simulink library "sm_motor_grader_lib"  (R2026a)
settings: Solver=VariableStepAuto
undefined symbols (not defined in the file): activeTestCmds, Art, Center, Circle, Driver, HMPST, LiftL, LiftR, LnL, LnR, Loads, Maneuver, motGradParams, Pin, RFL, RFR, RRL, RRR, SceneData, Side, Sphere, StrL, StrR, Tilt, X, Y, Z
libraries: sm_lib x219, nesl_utility x134, fl_lib x53, $bdroot x24, cvt_powertrain_lib x6, simulink_extras x5, grid_element x4, simulink x3, cvt_powertrain_lib_vnts x3, Driver_Long_Lat_Stanley x1, Maneuver_Get_Pose x1, SignalEditorBlockLib x1
(part 2 of 13)

== system sm_motor_grader_lib/Control ==
  m : Inport
  1-D Lookup Table : Lookup_n-D  NumberOfTableDimensions=1  BreakpointsForDimension1=activeTestCmds.get('pArtic').Time  Table=activeTestCmds.get('pArtic').Data  InternalRulePriority=Speed  RndMeth=Simplest
  1-D Lookup Table1 : Lookup_n-D  NumberOfTableDimensions=1  BreakpointsForDimension1=activeTestCmds.get('nHoleLink').Time  Table=activeTestCmds.get('nHoleLink').Data  InternalRulePriority=Speed  RndMeth=Simplest
  1-D Lookup Table10 : Lookup_n-D  NumberOfTableDimensions=1  BreakpointsForDimension1=activeTestCmds.get('qCircle').Time  Table=activeTestCmds.get('qCircle').Data  InternalRulePriority=Speed  RndMeth=Simplest
  1-D Lookup Table11 : Lookup_n-D  NumberOfTableDimensions=1  BreakpointsForDimension1=activeTestCmds.get('mLiftL').Time  Table=activeTestCmds.get('mLiftL').Data  InternalRulePriority=Speed  RndMeth=Simplest
  1-D Lookup Table12 : Lookup_n-D  NumberOfTableDimensions=1  BreakpointsForDimension1=activeTestCmds.get('pPin').Time  Table=activeTestCmds.get('pPin').Data  InternalRulePriority=Speed  RndMeth=Simplest
  1-D Lookup Table13 : Lookup_n-D  NumberOfTableDimensions=1  BreakpointsForDimension1=activeTestCmds.get('mLiftR').Time  Table=activeTestCmds.get('mLiftR').Data  InternalRulePriority=Speed  RndMeth=Simplest
  1-D Lookup Table2 : Lookup_n-D  NumberOfTableDimensions=1  BreakpointsForDimension1=activeTestCmds.get('vVeh').Time  Table=activeTestCmds.get('vVeh').Data  InternalRulePriority=Speed  RndMeth=Simplest
  1-D Lookup Table3 : Lookup_n-D  NumberOfTableDimensions=1  BreakpointsForDimension1=activeTestCmds.get('pSteer').Time  Table=activeTestCmds.get('pSteer').Data  InternalRulePriority=Speed  RndMeth=Simplest
  1-D Lookup Table4 : Lookup_n-D  NumberOfTableDimensions=1  BreakpointsForDimension1=activeTestCmds.get('pLean').Time  Table=activeTestCmds.get('pLean').Data  InternalRulePriority=Speed  RndMeth=Simplest
  1-D Lookup Table5 : Lookup_n-D  NumberOfTableDimensions=1  BreakpointsForDimension1=activeTestCmds.get('pLiftL').Time  Table=activeTestCmds.get('pLiftL').Data  InternalRulePriority=Speed  RndMeth=Simplest
  1-D Lookup Table6 : Lookup_n-D  NumberOfTableDimensions=1  BreakpointsForDimension1=activeTestCmds.get('pLiftR').Time  Table=activeTestCmds.get('pLiftR').Data  InternalRulePriority=Speed  RndMeth=Simplest
  1-D Lookup Table7 : Lookup_n-D  NumberOfTableDimensions=1  BreakpointsForDimension1=activeTestCmds.get('pCircleShift').Time  Table=activeTestCmds.get('pCircleShift').Data  InternalRulePriority=Speed  RndMeth=Simplest
  1-D Lookup Table8 : Lookup_n-D  NumberOfTableDimensions=1  BreakpointsForDimension1=activeTestCmds.get('pTilt').Time  Table=activeTestCmds.get('pTilt').Data  InternalRulePriority=Speed  RndMeth=Simplest
  1-D Lookup Table9 : Lookup_n-D  NumberOfTableDimensions=1  BreakpointsForDimension1=activeTestCmds.get('pShift').Time  Table=activeTestCmds.get('pShift').Data  InternalRulePriority=Speed  RndMeth=Simplest
  Bus Creator : BusCreator  Inputs=14
  Bus Selector : BusSelector  OutputSignals=aSteerWheel
  Clock : Clock
  Closed Loop : Subsystem  VariantControl=Closed_Loop
  Steer Wheel to Cyl Ext : Subsystem
  Terminator2 : Terminator
  Test : Outport
  wires:
  m/1 -> Closed Loop/1(VehBus)
  Closed Loop/1(DrvBus) -> Bus Selector/1
  1-D Lookup Table7/1 -> Bus Creator/7  "pCircleShift"
  1-D Lookup Table/1 -> Bus Creator/2, Steer Wheel to Cyl Ext/2(pArtic)  "pArtic"
  1-D Lookup Table1/1 -> Bus Creator/12  "nHoleLink"
  1-D Lookup Table9/1 -> Bus Creator/10  "pShift"
  1-D Lookup Table2/1 -> Bus Creator/1  "vVeh"
  1-D Lookup Table8/1 -> Bus Creator/9  "pTilt"
  1-D Lookup Table12/1 -> Bus Creator/11  "pPin"
  1-D Lookup Table4/1 -> Bus Creator/4  "pLean"
  1-D Lookup Table6/1 -> Bus Creator/6  "pLiftR"
  Clock/1 -> 1-D Lookup Table/1, 1-D Lookup Table3/1, 1-D Lookup Table6/1, 1-D Lookup Table7/1, 1-D Lookup Table10/1, 1-D Lookup Table8/1, 1-D Lookup Table12/1, 1-D Lookup Table13/1, 1-D Lookup Table11/1, 1-D Lookup Table1/1, 1-D Lookup Table9/1, 1-D Lookup Table5/1, 1-D Lookup Table4/1, 1-D Lookup Table2/1
  Bus Creator/1 -> Test/1
  1-D Lookup Table10/1 -> Bus Creator/8  "qCircle"
  1-D Lookup Table5/1 -> Bus Creator/5  "pLiftL"
  Bus Selector/1 -> Steer Wheel to Cyl Ext/1(qSteer)  "<aSteerWheel>"
  Steer Wheel to Cyl Ext/1(pSteer) -> Bus Creator/3  "pSteer"
  1-D Lookup Table3/1 -> Terminator2/1  "pSteer"
  1-D Lookup Table11/1 -> Bus Creator/13  "mLiftL"
  1-D Lookup Table13/1 -> Bus Creator/14  "mLiftR"

== system sm_motor_grader_lib/Dashboard Input ==
  In : Inport
  Rate Limiter : RateLimiter  RisingSlewLimit=abs((upper_bound-lower_bound)/5)  FallingSlewLimit=-abs((upper_bound-lower_bound)/5)  SampleTimeMode=inherited  InitialCondition=U0
  Saturation : Saturate  UpperLimit=upper_bound  LowerLimit=lower_bound  ZeroCross=off
  Transfer Fcn (with initial outputs) : simulink_extras/Additional Linear/Transfer Fcn (with initial outputs)  N=[1]  D="[tfilt  1]"  Y0=U0  U0=U0
  out : Outport
  wires:
  In/1 -> Saturation/1
  Transfer Fcn (with initial outputs)/1 -> Rate Limiter/1
  Saturation/1 -> Transfer Fcn (with initial outputs)/1
  Rate Limiter/1 -> out/1

== system sm_motor_grader_lib/Data ==
  note: Easy way to create structure for simulation data.
  m : Inport
  1-D Lookup Table : Lookup_n-D  NumberOfTableDimensions=1  BreakpointsForDimension1=activeTestCmds.get('pArtic').Time  Table=activeTestCmds.get('pArtic').Data  InternalRulePriority=Speed  RndMeth=Simplest
  1-D Lookup Table1 : Lookup_n-D  NumberOfTableDimensions=1  BreakpointsForDimension1=activeTestCmds.get('nHoleLink').Time  Table=activeTestCmds.get('nHoleLink').Data  InternalRulePriority=Speed  RndMeth=Simplest
  1-D Lookup Table10 : Lookup_n-D  NumberOfTableDimensions=1  BreakpointsForDimension1=activeTestCmds.get('qCircle').Time  Table=activeTestCmds.get('qCircle').Data  InternalRulePriority=Speed  RndMeth=Simplest
  1-D Lookup Table11 : Lookup_n-D  NumberOfTableDimensions=1  BreakpointsForDimension1=activeTestCmds.get('mLiftL').Time  Table=activeTestCmds.get('mLiftL').Data  InternalRulePriority=Speed  RndMeth=Simplest
  1-D Lookup Table12 : Lookup_n-D  NumberOfTableDimensions=1  BreakpointsForDimension1=activeTestCmds.get('pPin').Time  Table=activeTestCmds.get('pPin').Data  InternalRulePriority=Speed  RndMeth=Simplest
  1-D Lookup Table13 : Lookup_n-D  NumberOfTableDimensions=1  BreakpointsForDimension1=activeTestCmds.get('mLiftR').Time  Table=activeTestCmds.get('mLiftR').Data  InternalRulePriority=Speed  RndMeth=Simplest
  1-D Lookup Table2 : Lookup_n-D  NumberOfTableDimensions=1  BreakpointsForDimension1=activeTestCmds.get('vVeh').Time  Table=activeTestCmds.get('vVeh').Data  InternalRulePriority=Speed  RndMeth=Simplest
  1-D Lookup Table3 : Lookup_n-D  NumberOfTableDimensions=1  BreakpointsForDimension1=activeTestCmds.get('pSteer').Time  Table=activeTestCmds.get('pSteer').Data  InternalRulePriority=Speed  RndMeth=Simplest
  1-D Lookup Table4 : Lookup_n-D  NumberOfTableDimensions=1  BreakpointsForDimension1=activeTestCmds.get('pLean').Time  Table=activeTestCmds.get('pLean').Data  InternalRulePriority=Speed  RndMeth=Simplest
  1-D Lookup Table5 : Lookup_n-D  NumberOfTableDimensions=1  BreakpointsForDimension1=activeTestCmds.get('pLiftL').Time  Table=activeTestCmds.get('pLiftL').Data  InternalRulePriority=Speed  RndMeth=Simplest
  1-D Lookup Table6 : Lookup_n-D  NumberOfTableDimensions=1  BreakpointsForDimension1=activeTestCmds.get('pLiftR').Time  Table=activeTestCmds.get('pLiftR').Data  InternalRulePriority=Speed  RndMeth=Simplest
  1-D Lookup Table7 : Lookup_n-D  NumberOfTableDimensions=1  BreakpointsForDimension1=activeTestCmds.get('pCircleShift').Time  Table=activeTestCmds.get('pCircleShift').Data  InternalRulePriority=Speed  RndMeth=Simplest
  1-D Lookup Table8 : Lookup_n-D  NumberOfTableDimensions=1  BreakpointsForDimension1=activeTestCmds.get('pTilt').Time  Table=activeTestCmds.get('pTilt').Data  InternalRulePriority=Speed  RndMeth=Simplest
  1-D Lookup Table9 : Lookup_n-D  NumberOfTableDimensions=1  BreakpointsForDimension1=activeTestCmds.get('pShift').Time  Table=activeTestCmds.get('pShift').Data  InternalRulePriority=Speed  RndMeth=Simplest
  Bus Creator : BusCreator  Inputs=14
  Clock : Clock
  Signal Editor : SignalEditorBlockLib/Signal Editor  Commented=on  FileName=MotGradTestCommands.mat  ActiveScenario=TestCmds  ActiveSignal=nHoleLink  IsBus=off  OutputBusObjectStr=Bus: BusObject  SampleTime=0  Interpolate=off  ZeroCross=off  OutputAfterFinalValue=Setting to zero  Unit=inherit  PreserveSignalName=on  ApplySigPropsToAllScenarios=on  ApplySigPropsToAllSignals=off  SignalPropertySource=Dialog parameters
  Terminator : Terminator
  Transfer Fcn : TransferFcn  Denominator=[0.1 1]
  Test : Outport
  wires:
  Clock/1 -> 1-D Lookup Table9/1, 1-D Lookup Table12/1, 1-D Lookup Table13/1, 1-D Lookup Table11/1, 1-D Lookup Table1/1, 1-D Lookup Table8/1, 1-D Lookup Table10/1, 1-D Lookup Table7/1, 1-D Lookup Table6/1, 1-D Lookup Table5/1, 1-D Lookup Table4/1, 1-D Lookup Table3/1, 1-D Lookup Table/1, 1-D Lookup Table2/1
  1-D Lookup Table7/1 -> Bus Creator/7  "pCircleShift"
  1-D Lookup Table10/1 -> Bus Creator/8  "qCircle"
  1-D Lookup Table12/1 -> Bus Creator/11  "pPin"
  1-D Lookup Table1/1 -> Bus Creator/12  "nHoleLink"
  1-D Lookup Table4/1 -> Bus Creator/4  "pLean"
  1-D Lookup Table/1 -> Bus Creator/2  "pArtic"
  1-D Lookup Table5/1 -> Bus Creator/5  "pLiftL"
  1-D Lookup Table8/1 -> Bus Creator/9  "pTilt"
  1-D Lookup Table9/1 -> Bus Creator/10  "pShift"
  1-D Lookup Table3/1 -> Bus Creator/3  "pSteer"
  1-D Lookup Table6/1 -> Bus Creator/6  "pLiftR"
  Transfer Fcn/1 -> Bus Creator/1  "vVeh"
  Bus Creator/1 -> Test/1
  m/1 -> Terminator/1
  1-D Lookup Table11/1 -> Bus Creator/13  "mLiftL"
  1-D Lookup Table13/1 -> Bus Creator/14  "mLiftR"
  1-D Lookup Table2/1 -> Transfer Fcn/1  "vVeh"

== system sm_motor_grader_lib/Drawbar ==
  Bus Element In : Inport  PortName=cmd  Element=qCircle
  Actuator : Subsystem  Variant=on  VariantControlMode=label  VariantControl=Position  LabelModeActiveChoice=Position
      settings: AttributesFormatString=%<LabelModeActiveChoice>
  Common Gear Constraint : sm_lib/Gears and Couplings/Gears/Common Gear Constraint  GearType=Internal  SpecificationType=CenterDistanceRatio  CenterDistance=0.439843707288225  CenterDistanceUnits=m  GearRatio=25/3  BaseGearRadius=1  BaseGearRadiusUnits=m  FollGearRadius=1  FollGearRadiusUnits=m  SensingForceTorqueDirection=FollowerOnBase  SensingForceTorqueResolutionFrame=BaseFrame  SenseForce=off  SenseTorque=off
  Drawbar : Subsystem
      settings: PortSchema="{\"entries\":[{\"content\":{\"sides\":[{\"content\":{\"connectorIds\":[\"LConn1\",\"LConn2\",\"LConn3\"]},\"type\":\"ConnectorPlacement.EquallySpacedRectSide\",\"uuid\":\"c5f191b1-521e-4128-9ed3-e7d77db4b9ac\"},{\"content\":{\"connectorIds\":[\"RConn1\"],\"side\":\"RIGHT\"},\"type\":\"ConnectorPlacement.EquallySpacedRectSide\",\"uuid\":\"8d32ccf5-09eb-45be-b318-439daa2ebdec\"},{\"content\":{\"connectorIds\":[\"LConn4\",\"LConn5\"],\"side\":\"TOP\"},\"type\":\"ConnectorPlacement.EquallySpacedRectSide\",\"uuid\":\"7fd453ba-2af2-4d29-90fe-6a5fb43a17e4\"}]},\"type\":\"ConnectorPlacement.EquallySpacedConnector\",\"uuid\":\"3987b159-0399-4627-a491-adadc6044e15\"}],\"packageUris\":[\"http://schema.mathworks.com/mf0/Connector/R2020b\"],\"version\":\"1.0\"}"
      mask Display: image('sm_motor_grader_drawbar_IMAGE.png')
  Gain1 : Gain  Gain=motGradParams.circleRot.gearRatio
  Pinion Gear : Subsystem
      settings: PortSchema="{\"entries\":[{\"content\":{\"sides\":[{\"content\":{},\"type\":\"ConnectorPlacement.EquallySpacedRectSide\",\"uuid\":\"c603bcd7-3b50-4fd0-b707-575b3b9ab760\"},{\"content\":{\"connectorIds\":[\"RConn1\"],\"side\":\"RIGHT\"},\"type\":\"ConnectorPlacement.EquallySpacedRectSide\",\"uuid\":\"75766ee4-4855-409c-acb4-47e2457aa3e0\"},{\"content\":{\"connectorIds\":[\"LConn1\"],\"side\":\"TOP\"},\"type\":\"ConnectorPlacement.EquallySpacedRectSide\",\"uuid\":\"8e8e6d6f-405e-48e3-9dc6-817f2641e967\"}]},\"type\":\"ConnectorPlacement.EquallySpacedConnector\",\"uuid\":\"69d12768-35c2-4c56-b984-34512094e0a2\"}],\"packageUris\":[\"http://schema.mathworks.com/mf0/Connector/R2020b\"],\"version\":\"1.0\"}"
      mask Display: image('sm_motor_grader_pinion_IMAGE.png')
  Revolute Circle : Subsystem
  Spherical Frame : sm_lib/Joints/Spherical Joint  JointMode=Normal  CompositeWrenchDir=FollowerOnBase  CompositeWrenchFrame=BaseFrame  SenseConstraintForce=off  SenseConstraintTorque=off  SenseTotalForce=off  SenseTotalTorque=off  PositionTargetSpecify=on  PositionTargetPriority=Low  PositionTargetRotationMethod=AlignedAxes  PositionTargetFollAlignAxisA=+X  PositionTargetBaseAlignAxisA=+X  PositionTargetFollAlignAxisB=+Y  PositionTargetBaseAlignAxisB=+Y  PositionTargetRotationStandardAxis=+Z  PositionTargetRotationAngle=0  PositionTargetRotationAngleUnits=deg  PositionTargetRotationArbitraryAxis=[0 0 1]  PositionTargetRotationSequenceAxes=FollowerAxes  PositionTargetRotationSequence=XYX  PositionTargetRotationSequenceAngles=[0 0 0]  PositionTargetRotationSequenceAnglesUnits=deg  PositionTargetRotationMatrix=[1 0 0;0 1 0;0 0 1]  PositionTargetQuaternion=[1 0 0 0]  VelocityTargetSpecify=off  VelocityTargetPriority=High  VelocityTargetValue=[0 0 0]  VelocityTargetValueUnits=deg/s  VelocityTargetInFollowerFrame=on  EqPosRotationMethod=None  EqPosFollAlignAxisA=+X  EqPosBaseAlignAxisA=+Y  EqPosFollAlignAxisB=+Y  EqPosBaseAlignAxisB=+Z  EqPosRotationStandardAxis=+Z  EqPosRotationAngle=0  EqPosRotationAngleUnits=deg  EqPosRotationArbitraryAxis=[0 0 1]  EqPosRotationSequenceAxes=FollowerAxes  EqPosRotationSequence=XYX  EqPosRotationSequenceAngles=[0 0 0]  EqPosRotationSequenceAnglesUnits=deg  EqPosRotationMatrix=[1 0 0;0 1 0;0 0 1]  EqPosQuaternion=[1 0 0 0]  SpringStiffness=0  SpringStiffnessUnits=N*m/deg  DampingCoefficient=motGradParams.sphDampingCoeff  DampingCoefficientUnits=N*m/(deg/s)  LowerLimitSpecify=off  LowerLimitBound=15  LowerLimitBoundUnits=deg  LowerLimitStiffness=1e4  LowerLimitStiffnessUnits=N*m/deg  LowerLimitDamping=10  LowerLimitDampingUnits=N*m/(deg/s)  LowerLimitTransitionRegionWidth=0.1  LowerLimitTransitionRegionWidthUnits=deg  UpperLimitSpecify=off  UpperLimitBound=45  UpperLimitBoundUnits=deg  UpperLimitStiffness=1e4  UpperLimitStiffnessUnits=N*m/deg  UpperLimitDamping=10  UpperLimitDampingUnits=N*m/(deg/s)  UpperLimitTransitionRegionWidth=0.1  UpperLimitTransitionRegionWidthUnits=deg  TorqueActuationMode=NoTorque  ActuateTorqueX=off  ActuateTorqueY=off  ActuateTorqueZ=off  ActuateTorque=off  ActuationFrame=BaseFrame  SensePosition=off  SenseVelocityX=off  SenseVelocityY=off  SenseVelocityZ=off  SenseVelocity=off  SenseAccelerationX=off  SenseAccelerationY=off  SenseAccelerationZ=off  SenseAcceleration=off  SenseLowerLimitTorqueMag=off  SenseUpperLimitTorqueMag=off  SensingFrame=BaseFrame
  LiftL : PMIOPort  Side=Left
  LiftR : PMIOPort  Port=2  Side=Left
  Shift : PMIOPort  Port=3  Side=Left
  Frame : PMIOPort  Port=4  Side=Right
  Circle : PMIOPort  Port=5  Side=Right
  Pinion : PMIOPort  Port=6  Side=Right
  Out Bus Element : Outport  PortName=m  Element=Circle
  Out Bus Element1 : Outport  PortName=m  Element=Pinion
  wires:
  Bus Element In/1 -> Gain1/1
  Gain1/1 -> Actuator/1(q)
  Revolute Circle/1(m) -> Out Bus Element/1
  Actuator/1(m) -> Out Bus Element1/1
  connections:
  Frame/RConn1 -- Spherical Frame/LConn1
  Circle/RConn1 -- Common Gear Constraint/RConn1 -- Revolute Circle/RConn1
  Drawbar/LConn1 -- LiftL/RConn1
  Drawbar/LConn2 -- LiftR/RConn1
  Common Gear Constraint/LConn1 -- Pinion Gear/LConn1
  Actuator/RConn1 -- Pinion Gear/RConn1
  Pinion/RConn1 -- Actuator/LConn1
  Spherical Frame/RConn1 -- Drawbar/RConn1
  Revolute Circle/LConn1 -- Drawbar/LConn4
  Actuator/LConn2 -- Drawbar/LConn5
  Drawbar/LConn3 -- Shift/RConn1

== system sm_motor_grader_lib/Frame ==
  In Bus Element : Inport  PortName=cmd  Element=pPin
  Cab : Subsystem
      mask Display: image('sm_motor_grader_cab_IMAGE.png');
  Frame : Subsystem
      settings: PortSchema="{\"entries\":[{\"content\":{\"sides\":[{\"content\":{\"connectorIds\":[\"LConn1\",\"LConn2\",\"LConn3\"]},\"type\":\"ConnectorPlacement.EquallySpacedRectSide\",\"uuid\":\"3cc43cc8-f8b0-4e6c-bbf8-06577467423e\"},{\"content\":{\"connectorIds\":[\"RConn1\",\"RConn2\"],\"side\":\"RIGHT\"},\"type\":\"ConnectorPlacement.EquallySpacedRectSide\",\"uuid\":\"5e6794d0-63d3-423d-8b5c-0e3a6a58fbdc\"},{\"content\":{\"side\":\"TOP\"},\"type\":\"ConnectorPlacement.EquallySpacedRectSide\",\"uuid\":\"99c0f23c-f1a6-459b-839b-cf88b9a4fb05\"},{\"content\":{\"connectorIds\":[\"RConn3\",\"RConn4\",\"RConn5\"],\"side\":\"BOTTOM\"},\"type\":\"ConnectorPlacement.EquallySpacedRectSide\",\"uuid\":\"a57f33c3-f8fe-450e-b3de-9550f46fa3b6\"}]},\"type\":\"ConnectorPlacement.EquallySpacedConnector\",\"uuid\":\"81d8b758-f28c-4ca7-b27e-39357bec09b0\"}],\"packageUris\":[\"http://schema.mathworks.com/mf0/Connector/R2020b\"],\"version\":\"1.0\"}"
      mask Display: image('sm_motor_grader_frame_IMAGE.png')
  Prismatic Joint : sm_lib/Joints/Prismatic Joint  JointMode=Normal  CompositeWrenchDir=FollowerOnBase  CompositeWrenchFrame=BaseFrame  SenseConstraintForce=off  SenseConstraintTorque=off  SenseTotalForce=off  SenseTotalTorque=off  PositionTargetSpecify=off  PositionTargetPriority=High  PositionTargetValue=0  PositionTargetValueUnits=m  VelocityTargetSpecify=off  VelocityTargetPriority=High  VelocityTargetValue=0  VelocityTargetValueUnits=m/s  EquilibriumPosition=0  EquilibriumPositionUnits=m  SpringStiffness=0  SpringStiffnessUnits=N/m  DampingCoefficient=0  DampingCoefficientUnits=N/(m/s)  LowerLimitSpecify=off  LowerLimitBound=-0.1  LowerLimitBoundUnits=m  LowerLimitStiffness=1e2  LowerLimitStiffnessUnits=N/m  LowerLimitDamping=1e1  LowerLimitDampingUnits=N/(m/s)  LowerLimitTransitionRegionWidth=1e-2  LowerLimitTransitionRegionWidthUnits=m  UpperLimitSpecify=off  UpperLimitBound=0  UpperLimitBoundUnits=m  UpperLimitStiffness=1e2  UpperLimitStiffnessUnits=N/m  UpperLimitDamping=1e1  UpperLimitDampingUnits=N/(m/s)  UpperLimitTransitionRegionWidth=1e-2  UpperLimitTransitionRegionWidthUnits=m  TorqueActuationMode=ComputedTorque  MotionActuationMode=InputMotion  SensePosition=off  SenseVelocity=off  SenseAcceleration=off  SenseTorqueForce=off  SenseLowerLimitTorqueForce=off  SenseUpperLimitTorqueForce=off
  SaddlePinSolid : sm_lib/Body Elements/File Solid  ExtGeomFileName=SaddlePin.step  UnitType=FromFile  ExtGeomFileUnits=m  StepReaderType=HEX  ExportConvexHullGeometry=off  InertiaType=CalculateFromGeometry  BasedOnType=Mass  Density=1000  DensityUnits=kg/m^3  Mass=motGradParams.saddlePin.mass  MassUnits=kg  CenterOfMass=[0 0 0]  CenterOfMassUnits=m  MomentsOfInertia=[1 1 1]  MomentsOfInertiaUnits=kg*m^2  ProductsOfInertia=[0 0 0]  ProductsOfInertiaUnits=kg*m^2  GraphicType=FromGeometry  MarkerShape=Sphere  MarkerSize=10  GraphicVisPropType=SimpleVisualProperties  GraphicDiffuseColor=mtrgrd.clr.saddle_pin  GraphicOpacity=1  GraphicSpecularColor=[0.5 0.5 0.5 1.0]  GraphicAmbientColor=[0.15 0.15 0.15 1.0]  GraphicEmissiveColor=[0.0 0.0 0.0 1.0]  GraphicShininess=75  DoExposeReferenceFrame=off  SerializedFrames=<Frames><Frame><Id>Frame1</Id><Value><Name>MainFrame</Name><Origin><Source>GeometricFeature</Source><FeatureName>circular curve 2</FeatureName></Origin><PrimaryAxis><DefinedDirection>+Z</DefinedDirection><Source>GeometricFeature</Source><SourceDirection>+Z</SourceDirection><FeatureName>segment 1</FeatureName></PrimaryAxis><SecondaryAxis><DefinedDirection>+X</DefinedDirection><Source>ReferenceFrame</Source><SourceDirection>+X</SourceDirection><FeatureName></FeatureName></SecondaryAxis></Value></Frame><Frame><Id>Frame2</Id><Value><Name>LinkBar</Name><Origin><Source>GeometricFeature</Source><FeatureName>circular curve 4</FeatureName></Origin><PrimaryAxis><DefinedDirection>+Z</DefinedDirection><Source>GeometricFeature</Source><SourceDirection>+Z</SourceDirection><FeatureName>segment 1</FeatureName></PrimaryAxis><SecondaryAxis><DefinedDirection>+X</DefinedDirection><Source>ReferenceFrame</Source><SourceDirection>+X</SourceDirection><FeatureName></FeatureName></SecondaryAxis></Value></Frame></Frames>
  Simulink-PS Converter : nesl_utility/Simulink-PS Converter  PhysicalDomain=network_engine_domain  SubClassName=ps_input  LeftPortType=input  RightPortType=output  PseudoPeriodic=off  Frequencies=[]  NoiseDistribution=none  NoiseParameters=[]  Unit=m  AffineConversion=off  FilteringAndDerivatives=filter  SimscapeFilterOrder=2  InputFilterTimeConstant=0.001  UdotUserProvided=0
  Cyl : PMIOPort  Side=Left
  R : PMIOPort  Port=2  Side=Left
  F : PMIOPort  Port=3  Side=Right
  Drawbar : PMIOPort  Port=4  Side=Right
  SaddleL : PMIOPort  Port=5  Side=Right
  LinkBar : PMIOPort  Port=6  Side=Right
  SaddleR : PMIOPort  Port=7  Side=Right
  LinkBar1 : PMIOPort  Port=8  Side=Right
  LinkBar2 : PMIOPort  Port=9  Side=Right
  LinkBar3 : PMIOPort  Port=10  Side=Right
  wires:
  In Bus Element/1 -> Simulink-PS Converter/1
  connections:
  LinkBar/RConn1 -- LinkBar1/RConn1 -- LinkBar2/RConn1 -- LinkBar3/RConn1 -- SaddlePinSolid/RConn1
  SaddlePinSolid/LConn1 -- Prismatic Joint/RConn1
  Simulink-PS Converter/RConn1 -- Prismatic Joint/LConn2
  Drawbar/RConn1 -- Frame/RConn1
  Frame/RConn2 -- F/RConn1
  Frame/LConn2 -- Cyl/RConn1
  R/RConn1 -- Frame/LConn3
  Cab/RConn1 -- Frame/LConn1
  Frame/RConn3 -- SaddleL/RConn1
  SaddleR/RConn1 -- Frame/RConn5
  Prismatic Joint/LConn1 -- Frame/RConn4

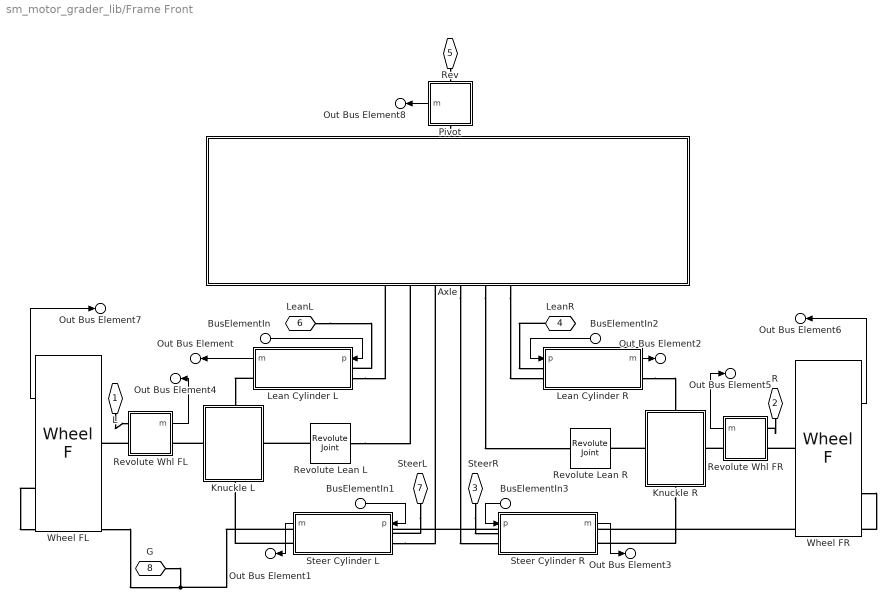
== system sm_motor_grader_lib/Frame Front ==
  BusElementIn : Inport  PortName=cmd  Element=pLeanL
  BusElementIn1 : Inport  PortName=cmd  Element=pSteerL
  BusElementIn2 : Inport  PortName=cmd  Element=pLeanR
  BusElementIn3 : Inport  PortName=cmd  Element=pSteerR
  Axle : Subsystem
      mask Display: image('sm_motor_grader_axleF_IMAGE.png');
  Knuckle L : Subsystem
      settings: PortSchema="{\"entries\":[{\"content\":{\"sides\":[{\"content\":{\"connectorIds\":[\"LConn1\"]},\"type\":\"ConnectorPlacement.EquallySpacedRectSide\",\"uuid\":\"76f50f5e-04f6-4db5-a4c2-d2b97709e12f\"},{\"content\":{\"connectorIds\":[\"RConn1\"],\"side\":\"RIGHT\"},\"type\":\"ConnectorPlacement.EquallySpacedRectSide\",\"uuid\":\"b3c1357e-70d1-41c6-bb27-3450430a84f7\"},{\"content\":{\"connectorIds\":[\"LConn2\"],\"side\":\"TOP\"},\"type\":\"ConnectorPlacement.EquallySpacedRectSide\",\"uuid\":\"226f928b-a182-43a4-8a68-f5ff8d6ac951\"},{\"content\":{\"connectorIds\":[\"RConn2\"],\"side\":\"BOTTOM\"},\"type\":\"ConnectorPlacement.EquallySpacedRectSide\",\"uuid\":\"a8a8e93d-d06d-4136-a56a-52642eb3b6bf\"}]},\"type\":\"ConnectorPlacement.EquallySpacedConnector\",\"uuid\":\"6e5a9dc5-0e8d-434d-bc69-c9fce24e87db\"}],\"packageUris\":[\"http://schema.mathworks.com/mf0/Connector/R2020b\"],\"version\":\"1.0\"}"
      mask Display: image('sm_motor_grader_knuckle_IMAGE.png');
  Knuckle R : Subsystem
      settings: PortSchema="{\"entries\":[{\"content\":{\"sides\":[{\"content\":{\"connectorIds\":[\"LConn1\"]},\"type\":\"ConnectorPlacement.EquallySpacedRectSide\",\"uuid\":\"76f50f5e-04f6-4db5-a4c2-d2b97709e12f\"},{\"content\":{\"connectorIds\":[\"RConn1\"],\"side\":\"RIGHT\"},\"type\":\"ConnectorPlacement.EquallySpacedRectSide\",\"uuid\":\"b3c1357e-70d1-41c6-bb27-3450430a84f7\"},{\"content\":{\"connectorIds\":[\"LConn2\"],\"side\":\"TOP\"},\"type\":\"ConnectorPlacement.EquallySpacedRectSide\",\"uuid\":\"226f928b-a182-43a4-8a68-f5ff8d6ac951\"},{\"content\":{\"connectorIds\":[\"RConn2\"],\"side\":\"BOTTOM\"},\"type\":\"ConnectorPlacement.EquallySpacedRectSide\",\"uuid\":\"3e5dcdd0-7ec1-4db4-9a17-a23d273abb04\"}]},\"type\":\"ConnectorPlacement.EquallySpacedConnector\",\"uuid\":\"6e5a9dc5-0e8d-434d-bc69-c9fce24e87db\"}],\"packageUris\":[\"http://schema.mathworks.com/mf0/Connector/R2020b\"],\"version\":\"1.0\"}"
      mask Display: image('sm_motor_grader_knuckle_IMAGE.png')
  Lean Cylinder L : Subsystem  mask{popup_actuator_model=Shaft}
      mask prompts: popup_actuator_model "Actuation Mode"
      mask init: same as sm_motor_grader_lib/Drawbar
      settings: AttributesFormatString=%<popup_actuator_model>
      mask TypeOptions popup_actuator_model: Position | Shaft
      mask Display:
      | bh = gcb;
      | if(strcmp(get_param(bh,'popup_actuator_model'),'Position'))
      |     image('sm_motor_grader_actuator_intfPosition_IMAGE.png')
      | else
      |     image('sm_motor_grader_actuator_intfShaft_IMAGE.png')
      | end
  Lean Cylinder R : Subsystem  mask{popup_actuator_model=Shaft}
      mask prompts: popup_actuator_model "Actuation Mode"
      mask init: same as sm_motor_grader_lib/Drawbar
      settings: AttributesFormatString=%<popup_actuator_model>
      mask TypeOptions popup_actuator_model: Position | Shaft
      mask Display:
      | bh = gcb;
      | if(strcmp(get_param(bh,'popup_actuator_model'),'Position'))
      |     image('sm_motor_grader_actuator_intfPosition_IMAGE.png')
      | else
      |     image('sm_motor_grader_actuator_intfShaft_IMAGE.png')
      | end
  Pivot : Subsystem
      settings: PortSchema="{\"entries\":[{\"content\":{\"sides\":[{\"content\":{\"connectorIds\":[\"LConn1\"]},\"type\":\"ConnectorPlacement.EquallySpacedRectSide\",\"uuid\":\"c9e5bf41-3876-4983-8e0e-21f1173e0e13\"},{\"content\":{\"connectorIds\":[\"RConn1\"],\"side\":\"RIGHT\"},\"type\":\"ConnectorPlacement.EquallySpacedRectSide\",\"uuid\":\"17d0e604-72cc-45c0-9bd2-f261f6cea6bf\"},{\"content\":{\"connectorIds\":[\"Out1\"],\"side\":\"TOP\"},\"type\":\"ConnectorPlacement.EquallySpacedRectSide\",\"uuid\":\"317782e4-d40b-4965-bfb3-1602ce258838\"}]},\"type\":\"ConnectorPlacement.EquallySpacedConnector\",\"uuid\":\"ff22ddf5-aef8-4561-9b08-81701ca29e49\"}],\"packageUris\":[\"http://schema.mathworks.com/mf0/Connector/R2020b\"],\"version\":\"1.0\"}"
  Revolute Whl FL : Subsystem
  Revolute Whl FR : Subsystem
  Revolute Lean L : sm_lib/Joints/Revolute Joint  JointMode=Normal  CompositeWrenchDir=FollowerOnBase  CompositeWrenchFrame=BaseFrame  SenseConstraintForce=off  SenseConstraintTorque=off  SenseTotalForce=off  SenseTotalTorque=off  PositionTargetSpecify=off  PositionTargetPriority=High  PositionTargetValue=0  PositionTargetValueUnits=deg  VelocityTargetSpecify=off  VelocityTargetPriority=High  VelocityTargetValue=0  VelocityTargetValueUnits=deg/s  EquilibriumPosition=0  EquilibriumPositionUnits=deg  SpringStiffness=0  SpringStiffnessUnits=N*m/deg  DampingCoefficient=0  DampingCoefficientUnits=N*m/(deg/s)  LowerLimitSpecify=off  LowerLimitBound=-90  LowerLimitBoundUnits=deg  LowerLimitStiffness=1e4  LowerLimitStiffnessUnits=N*m/deg  LowerLimitDamping=10  LowerLimitDampingUnits=N*m/(deg/s)  LowerLimitTransitionRegionWidth=0.1  LowerLimitTransitionRegionWidthUnits=deg  UpperLimitSpecify=off  UpperLimitBound=90  UpperLimitBoundUnits=deg  UpperLimitStiffness=1e4  UpperLimitStiffnessUnits=N*m/deg  UpperLimitDamping=10  UpperLimitDampingUnits=N*m/(deg/s)  UpperLimitTransitionRegionWidth=0.1  UpperLimitTransitionRegionWidthUnits=deg  TorqueActuationMode=NoTorque  MotionActuationMode=ComputedMotion  SensePosition=off  SenseVelocity=off  SenseAcceleration=off  SenseTorqueForce=off  SenseLowerLimitTorqueForce=off  SenseUpperLimitTorqueForce=off
  Revolute Lean R : sm_lib/Joints/Revolute Joint  JointMode=Normal  CompositeWrenchDir=FollowerOnBase  CompositeWrenchFrame=BaseFrame  SenseConstraintForce=off  SenseConstraintTorque=off  SenseTotalForce=off  SenseTotalTorque=off  PositionTargetSpecify=off  PositionTargetPriority=High  PositionTargetValue=0  PositionTargetValueUnits=deg  VelocityTargetSpecify=off  VelocityTargetPriority=High  VelocityTargetValue=0  VelocityTargetValueUnits=deg/s  EquilibriumPosition=0  EquilibriumPositionUnits=deg  SpringStiffness=0  SpringStiffnessUnits=N*m/deg  DampingCoefficient=0  DampingCoefficientUnits=N*m/(deg/s)  LowerLimitSpecify=off  LowerLimitBound=-90  LowerLimitBoundUnits=deg  LowerLimitStiffness=1e4  LowerLimitStiffnessUnits=N*m/deg  LowerLimitDamping=10  LowerLimitDampingUnits=N*m/(deg/s)  LowerLimitTransitionRegionWidth=0.1  LowerLimitTransitionRegionWidthUnits=deg  UpperLimitSpecify=off  UpperLimitBound=90  UpperLimitBoundUnits=deg  UpperLimitStiffness=1e4  UpperLimitStiffnessUnits=N*m/deg  UpperLimitDamping=10  UpperLimitDampingUnits=N*m/(deg/s)  UpperLimitTransitionRegionWidth=0.1  UpperLimitTransitionRegionWidthUnits=deg  TorqueActuationMode=NoTorque  MotionActuationMode=ComputedMotion  SensePosition=off  SenseVelocity=off  SenseAcceleration=off  SenseTorqueForce=off  SenseLowerLimitTorqueForce=off  SenseUpperLimitTorqueForce=off
  Steer Cylinder L : Subsystem  mask{popup_actuator_model=Shaft}
      mask prompts: popup_actuator_model "Actuation Mode"
      mask init: same as sm_motor_grader_lib/Drawbar
      settings: AttributesFormatString=%<popup_actuator_model>
      mask TypeOptions popup_actuator_model: Position | Shaft
      mask Display:
      | bh = gcb;
      | if(strcmp(get_param(bh,'popup_actuator_model'),'Position'))
      |     image('sm_motor_grader_actuator_intfPosition_IMAGE.png')
      | else
      |     image('sm_motor_grader_actuator_intfShaft_IMAGE.png')
      | end
  Steer Cylinder R : Subsystem  mask{popup_actuator_model=Shaft}
      mask prompts: popup_actuator_model "Actuation Mode"
      mask init: same as sm_motor_grader_lib/Drawbar
      settings: AttributesFormatString=%<popup_actuator_model>
      mask TypeOptions popup_actuator_model: Position | Shaft
      mask Display:
      | bh = gcb;
      | if(strcmp(get_param(bh,'popup_actuator_model'),'Position'))
      |     image('sm_motor_grader_actuator_intfPosition_IMAGE.png')
      | else
      |     image('sm_motor_grader_actuator_intfShaft_IMAGE.png')
      | end
  Wheel FL : $bdroot/Wheel F  popup_ground_contact=Sphere  popup_leftright=Left
  Wheel FR : $bdroot/Wheel F  popup_ground_contact=Sphere  popup_leftright=Right
  L : PMIOPort  Side=Left
  R : PMIOPort  Port=2  Side=Left
  SteerR : PMIOPort  Port=3  Side=Left
  LeanR : PMIOPort  Port=4  Side=Left
  Rev : PMIOPort  Port=5  Side=Left
  LeanL : PMIOPort  Port=6  Side=Left
  SteerL : PMIOPort  Port=7  Side=Left
  G : PMIOPort  Port=8  Side=Right
  Out Bus Element : Outport  PortName=m  Element=LeanL
  Out Bus Element1 : Outport  PortName=m  Element=SteerL
  Out Bus Element2 : Outport  PortName=m  Element=LeanR
  Out Bus Element3 : Outport  PortName=m  Element=SteerR
  Out Bus Element4 : Outport  PortName=m  Element=WhlL
  Out Bus Element5 : Outport  PortName=m  Element=WhlR
  Out Bus Element6 : Outport  PortName=m  Element=TireFR
  Out Bus Element7 : Outport  PortName=m  Element=TireFL
  Out Bus Element8 : Outport  PortName=m  Element=Pivot
  wires:
  BusElementIn/1 -> Lean Cylinder L/1(p)
  BusElementIn1/1 -> Steer Cylinder L/1(p)
  BusElementIn2/1 -> Lean Cylinder R/1(p)
  BusElementIn3/1 -> Steer Cylinder R/1(p)
  Lean Cylinder L/1(m) -> Out Bus Element/1
  Steer Cylinder L/1(m) -> Out Bus Element1/1
  Lean Cylinder R/1(m) -> Out Bus Element2/1
  Steer Cylinder R/1(m) -> Out Bus Element3/1
  Revolute Whl FL/1(m) -> Out Bus Element4/1
  Revolute Whl FR/1(m) -> Out Bus Element5/1
  Wheel FR/1 -> Out Bus Element6/1
  Wheel FL/1 -> Out Bus Element7/1
  Pivot/1(m) -> Out Bus Element8/1
  connections:
  G/RConn1 -- Wheel FR/RConn1 -- Wheel FL/RConn1
  Lean Cylinder R/RConn1 -- Knuckle R/LConn2
  Knuckle R/RConn1 -- Revolute Lean R/RConn1
  Revolute Whl FR/RConn1 -- Knuckle R/LConn1
  Revolute Lean L/RConn1 -- Knuckle L/RConn1
  Knuckle L/LConn1 -- Revolute Whl FL/RConn1
  Lean Cylinder L/LConn2 -- Axle/LConn7
  Steer Cylinder L/LConn2 -- Axle/LConn9
  Knuckle R/RConn2 -- Steer Cylinder R/RConn1
  Revolute Lean L/LConn1 -- Axle/LConn8
  Axle/LConn11 -- Revolute Lean R/LConn1
  Revolute Whl FL/LConn2 -- Wheel FL/LConn1
  Wheel FR/LConn1 -- Revolute Whl FR/LConn2
  Lean Cylinder L/RConn1 -- Knuckle L/LConn2
  Steer Cylinder L/RConn1 -- Knuckle L/RConn2
  Axle/LConn12 -- Lean Cylinder R/LConn2
  Axle/LConn10 -- Steer Cylinder R/LConn2
  LeanL/RConn1 -- Lean Cylinder L/LConn1
  SteerL/RConn1 -- Steer Cylinder L/LConn1
  LeanR/RConn1 -- Lean Cylinder R/LConn1
  SteerR/RConn1 -- Steer Cylinder R/LConn1
  L/RConn1 -- Revolute Whl FL/LConn1
  R/RConn1 -- Revolute Whl FR/LConn1
  Rev/RConn1 -- Pivot/RConn1
  Pivot/LConn1 -- Axle/RConn1

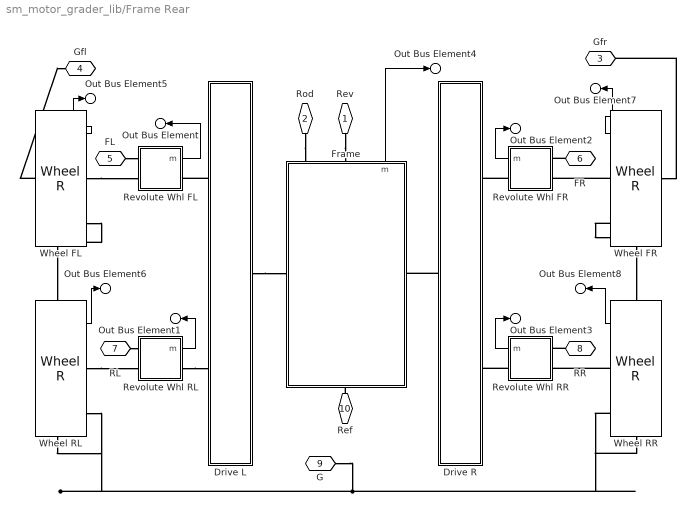
== system sm_motor_grader_lib/Frame Rear ==
  Drive L : Subsystem
  Drive R : Subsystem
  Frame : Subsystem
      settings: PortSchema="{\"entries\":[{\"content\":{\"sides\":[{\"content\":{\"connectorIds\":[\"LConn1\"]},\"type\":\"ConnectorPlacement.EquallySpacedRectSide\",\"uuid\":\"910fc5c3-2ac6-40fd-9a77-2a65450dab50\"},{\"content\":{\"connectorIds\":[\"RConn1\",\"RConn2\",\"Out1\"],\"side\":\"RIGHT\"},\"type\":\"ConnectorPlacement.EquallySpacedRectSide\",\"uuid\":\"832f97d3-ea25-499f-8919-fc7b6c585ebe\"},{\"content\":{\"connectorIds\":[\"LConn2\"],\"side\":\"TOP\"},\"type\":\"ConnectorPlacement.EquallySpacedRectSide\",\"uuid\":\"874b5af6-cc1c-4c18-b595-8474f21eb5dc\"},{\"content\":{\"connectorIds\":[\"RConn3\"],\"side\":\"BOTTOM\"},\"type\":\"ConnectorPlacement.EquallySpacedRectSide\",\"uuid\":\"384a01e6-481a-4670-b8ff-9da4ad195e93\"}]},\"type\":\"ConnectorPlacement.EquallySpacedConnector\",\"uuid\":\"5bf4ebed-69b2-4bdb-9bd3-6f78dc235d29\"}],\"packageUris\":[\"http://schema.mathworks.com/mf0/Connector/R2020b\"],\"version\":\"1.0\"}"
      mask Display: image('sm_motor_grader_frameRearHousing_IMAGE.png')
  Revolute Whl FL : Subsystem
  Revolute Whl FR : Subsystem
  Revolute Whl RL : Subsystem
  Revolute Whl RR : Subsystem
  Wheel FL : $bdroot/Wheel R  popup_ground_contact=Sphere  popup_leftright=Left
  Wheel FR : $bdroot/Wheel R  popup_ground_contact=Sphere  popup_leftright=Right
  Wheel RL : $bdroot/Wheel R  popup_ground_contact=Sphere  popup_leftright=Left
  Wheel RR : $bdroot/Wheel R  popup_ground_contact=Sphere  popup_leftright=Right
  Rev : PMIOPort  Side=Left
  Rod : PMIOPort  Port=2  Side=Left
  Gfr : PMIOPort  Port=3  Side=Right
  Gfl : PMIOPort  Port=4  Side=Right
  FL : PMIOPort  Port=5  Side=Right
  FR : PMIOPort  Port=6  Side=Right
  RL : PMIOPort  Port=7  Side=Right
  RR : PMIOPort  Port=8  Side=Right
  G : PMIOPort  Port=9  Side=Right
  Ref : PMIOPort  Port=10  Side=Right
  Out Bus Element : Outport  PortName=m  Element=WhlFL
  Out Bus Element1 : Outport  PortName=m  Element=WhlRL
  Out Bus Element2 : Outport  PortName=m  Element=WhlFR
  Out Bus Element3 : Outport  PortName=m  Element=WhlRR
  Out Bus Element4 : Outport  PortName=m  Element=Body
  Out Bus Element5 : Outport  PortName=m  Element=TireFL
  Out Bus Element6 : Outport  PortName=m  Element=TireRL
  Out Bus Element7 : Outport  PortName=m  Element=TireFR
  Out Bus Element8 : Outport  PortName=m  Element=TireRR
  wires:
  Revolute Whl FL/1(m) -> Out Bus Element/1
  Revolute Whl RL/1(m) -> Out Bus Element1/1
  Revolute Whl FR/1(m) -> Out Bus Element2/1
  Revolute Whl RR/1(m) -> Out Bus Element3/1
  Frame/1(m) -> Out Bus Element4/1
  Wheel FL/1 -> Out Bus Element5/1
  Wheel RL/1 -> Out Bus Element6/1
  Wheel FR/1 -> Out Bus Element7/1
  Wheel RR/1 -> Out Bus Element8/1
  connections:
  Rev/RConn1 -- Frame/RConn2
  Drive R/LConn1 -- Frame/RConn3
  Rod/RConn1 -- Frame/RConn1
  Drive L/RConn1 -- Frame/LConn2
  Ref/RConn1 -- Frame/LConn1
  Wheel FR/RConn1 -- Revolute Whl FR/LConn2
  Revolute Whl FR/RConn1 -- Drive R/RConn1
  Revolute Whl RR/RConn1 -- Drive R/RConn2
  Wheel RR/RConn1 -- Revolute Whl RR/LConn2
  G/RConn1 -- Wheel FR/RConn2 -- Wheel RR/RConn2 -- Wheel FL/RConn2 -- Wheel RL/RConn2
  Revolute Whl RL/RConn1 -- Drive L/LConn2
  Wheel RL/RConn1 -- Revolute Whl RL/LConn2
  Drive L/LConn1 -- Revolute Whl FL/RConn1
  Wheel FL/RConn1 -- Revolute Whl FL/LConn2
  FL/RConn1 -- Revolute Whl FL/LConn1
  RL/RConn1 -- Revolute Whl RL/LConn1
  FR/RConn1 -- Revolute Whl FR/LConn1
  RR/RConn1 -- Revolute Whl RR/LConn1
  Wheel FL/LConn1 -- Gfl/RConn1
  Wheel FR/LConn1 -- Gfr/RConn1

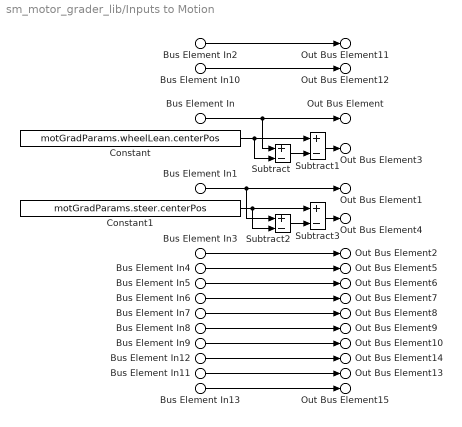
== system sm_motor_grader_lib/Inputs to Motion ==
  Bus Element In : Inport  PortName=Test  Element=pLean
  Bus Element In1 : Inport  PortName=Test  Element=pSteer
  Bus Element In2 : Inport  PortName=Test  Element=vVeh
  Bus Element In3 : Inport  PortName=Test  Element=pArtic
  Bus Element In4 : Inport  PortName=Test  Element=pLiftL
  Bus Element In5 : Inport  PortName=Test  Element=pLiftR
  Bus Element In6 : Inport  PortName=Test  Element=pCircleShift
  Bus Element In7 : Inport  PortName=Test  Element=qCircle
  Bus Element In8 : Inport  PortName=Test  Element=pTilt
  Bus Element In9 : Inport  PortName=Test  Element=pShift
  Bus Element In10 : Inport  PortName=Test  Element=nHoleLink
  Bus Element In12 : Inport  PortName=Test  Element=pPin
  Bus Element In11 : Inport  PortName=Test  Element=mLiftL
  Bus Element In13 : Inport  PortName=Test  Element=mLiftR
  Constant : Constant  Value=motGradParams.wheelLean.centerPos
  Constant1 : Constant  Value=motGradParams.steer.centerPos
  Subtract{,1..3} (4 alike) : Sum  Inputs=+-
  Out Bus Element : Outport  PortName=cmd  Element=pLeanL
  Out Bus Element1 : Outport  PortName=cmd  Element=pSteerL
  Out Bus Element2 : Outport  PortName=cmd  Element=pArtic
  Out Bus Element3 : Outport  PortName=cmd  Element=pLeanR
  Out Bus Element4 : Outport  PortName=cmd  Element=pSteerR
  Out Bus Element5 : Outport  PortName=cmd  Element=pLiftL
  Out Bus Element6 : Outport  PortName=cmd  Element=pLiftR
  Out Bus Element7 : Outport  PortName=cmd  Element=pCircleShift
  Out Bus Element8 : Outport  PortName=cmd  Element=qCircle
  Out Bus Element9 : Outport  PortName=cmd  Element=pTilt
  Out Bus Element10 : Outport  PortName=cmd  Element=pShift
  Out Bus Element11 : Outport  PortName=cmd  Element=vVeh
  Out Bus Element12 : Outport  PortName=cmd  Element=nHoleLink
  Out Bus Element14 : Outport  PortName=cmd  Element=pPin
  Out Bus Element13 : Outport  PortName=cmd  Element=mLiftL
  Out Bus Element15 : Outport  PortName=cmd  Element=mLiftR
  wires:
  Bus Element In/1 -> Subtract/1, Out Bus Element/1
  Subtract1/1 -> Out Bus Element3/1
  Subtract3/1 -> Out Bus Element4/1
  Subtract/1 -> Subtract1/2
  Bus Element In1/1 -> Subtract2/1, Out Bus Element1/1
  Constant/1 -> Subtract/2, Subtract1/1
  Subtract2/1 -> Subtract3/2
  Constant1/1 -> Subtract2/2, Subtract3/1
  Bus Element In2/1 -> Out Bus Element11/1
  Bus Element In3/1 -> Out Bus Element2/1
  Bus Element In4/1 -> Out Bus Element5/1
  Bus Element In5/1 -> Out Bus Element6/1
  Bus Element In6/1 -> Out Bus Element7/1
  Bus Element In7/1 -> Out Bus Element8/1
  Bus Element In8/1 -> Out Bus Element9/1
  Bus Element In9/1 -> Out Bus Element10/1
  Bus Element In10/1 -> Out Bus Element12/1
  Bus Element In12/1 -> Out Bus Element14/1
  Bus Element In13/1 -> Out Bus Element15/1
  Bus Element In11/1 -> Out Bus Element13/1

== system sm_motor_grader_lib/LiftAssembly ==
  Bus Element In{,1..3} (4 alike) : Inport  PortName=cmd
  Circle Shift : Subsystem  mask{popup_actuator_model=Shaft}
      mask prompts: popup_actuator_model "Actuation Mode"
      mask init: same as sm_motor_grader_lib/Drawbar
      settings: AttributesFormatString=%<popup_actuator_model>
      mask TypeOptions popup_actuator_model: Position | Shaft
      mask Display:
      | bh = gcb;
      | if(strcmp(get_param(bh,'popup_actuator_model'),'Position'))
      |     image('sm_motor_grader_actuator_intfPosition_IMAGE.png')
      | else
      |     image('sm_motor_grader_actuator_intfShaft_IMAGE.png')
      | end
  LinkBar : Subsystem  mask{popup_initial_hole=Center}
      mask prompts: popup_initial_hole "Initial Hole"
      mask init:
      | bh = gcb;
      | set_param([bh '/Left 3/Bushing'],...
      |     'PxPositionTargetSpecify','off','PyPositionTargetSpecify','off');
      | set_param([bh '/Left 2/Bushing'],...
      |     'PxPositionTargetSpecify','off','PyPositionTargetSpecify','off');
      | set_param([bh '/Left 1/Bushing'],...
      |     'PxPositionTargetSpecify','off','PyPositionTargetSpecify','off');
      | set_param([bh '/Center/Bushing'],...
      |     'PxPositionTargetSpecify','off','PyPositionTargetSpecify','off');
      | set_param([bh '/Right 1/Bushing'],...
      |     'PxPositionTargetSpecify','off','PyPositionTargetSpecify','off');
      | set_param([bh '/Right 2/Bushing'],...
      |     'PxPositionTargetSpecify','off','PyPositionTargetSpecify','off');
      | set_param([bh '/Right 3/Bushing'],...
      |     'PxPositionTargetSpecify','off','PyPositionTargetSpecify','off');
      | 
      | name_init_hole = get_param(bh,'popup_initial_hole');
      | set_param([bh '/' name_init_hole  '/Bushing'],...
      |     'PxPositionTargetSpecify','on','PyPositionTargetSpecify','on');
      settings: PortSchema="{\"entries\":[{\"content\":{\"sides\":[{\"content\":{\"connectorIds\":[\"LConn1\"]},\"type\":\"ConnectorPlacement.EquallySpacedRectSide\",\"uuid\":\"1c32e15d-523a-4644-9768-ca09a0f7e34b\"},{\"content\":{\"connectorIds\":[\"RConn1\"],\"side\":\"RIGHT\"},\"type\":\"ConnectorPlacement.EquallySpacedRectSide\",\"uuid\":\"3429a1cd-2c1c-42d1-8a06-de904a7192ad\"},{\"content\":{\"connectorIds\":[\"LConn2\"],\"side\":\"TOP\"},\"type\":\"ConnectorPlacement.EquallySpacedRectSide\",\"uuid\":\"4c4cca51-c1bd-4abb-8167-b36a18a8231a\"},{\"content\":{\"connectorIds\":[\"Out1\",\"In1\"],\"side\":\"BOTTOM\"},\"type\":\"ConnectorPlacement.EquallySpacedRectSide\",\"uuid\":\"38a263b0-df67-4637-9fc7-27a491e939a0\"}]},\"type\":\"ConnectorPlacement.EquallySpacedConnector\",\"uuid\":\"487e1662-4b24-45de-8fe4-1656aa9f1267\"}],\"packageUris\":[\"http://schema.mathworks.com/mf0/Connector/R2020b\"],\"version\":\"1.0\"}"
      mask TypeOptions popup_initial_hole: Left 3 | Left 2 | Left 1 | Center | Right 1 | Right 2 | Right 3
      mask Display: image('sm_motor_grader_linkbar_IMAGE.png')
  Saddle L : Subsystem  mask{popup_actuator_model=Shaft}
      mask prompts: popup_actuator_model "Actuation Mode"
      mask init: same as sm_motor_grader_lib/Drawbar
      settings: AttributesFormatString=%<popup_actuator_model>  PortSchema="{\"entries\":[{\"content\":{\"sides\":[{\"content\":{\"connectorIds\":[\"In1\",\"LConn1\",\"LConn2\"]},\"type\":\"ConnectorPlacement.EquallySpacedRectSide\",\"uuid\":\"d315f103-e951-475d-8879-0df00f385ed3\"},{\"content\":{\"connectorIds\":[\"Out1\",\"RConn1\",\"RConn2\"],\"side\":\"RIGHT\"},\"type\":\"ConnectorPlacement.EquallySpacedRectSide\",\"uuid\":\"e6a97a31-da14-4ed9-b748-a052924d916a\"},{\"content\":{\"side\":\"TOP\"},\"type\":\"ConnectorPlacement.EquallySpacedRectSide\",\"uuid\":\"8662f8b5-6fd1-48bd-b06f-ed035cdf755c\"},{\"content\":{\"connectorIds\":[\"RConn3\"],\"side\":\"BOTTOM\"},\"type\":\"ConnectorPlacement.EquallySpacedRectSide\",\"uuid\":\"773560ee-e149-4664-8312-786a14263625\"}]},\"type\":\"ConnectorPlacement.EquallySpacedConnector\",\"uuid\":\"22018313-0faf-46e6-b749-3ff6200247d9\"}],\"packageUris\":[\"http://schema.mathworks.com/mf0/Connector/R2020b\"],\"version\":\"1.0\"}"
      mask TypeOptions popup_actuator_model: Position | Shaft
      mask Display: image('sm_motor_grader_liftCylL_IMAGE.png')
  Saddle R : Subsystem  mask{popup_actuator_model=Shaft}
      mask prompts: popup_actuator_model "Actuation Mode"
      mask init: same as sm_motor_grader_lib/Drawbar
      settings: AttributesFormatString=%<popup_actuator_model>
      mask TypeOptions popup_actuator_model: Position | Shaft
      mask Display: image('sm_motor_grader_liftCylR_IMAGE.png');
  LiftLR : PMIOPort  Side=Left
  LiftRR : PMIOPort  Port=2  Side=Left
  Circle : PMIOPort  Port=3  Side=Left
  FrameL : PMIOPort  Port=4  Side=Left
  Pin : PMIOPort  Port=5  Side=Left
  FrameR : PMIOPort  Port=6  Side=Left
  LiftL : PMIOPort  Port=7  Side=Right
  LiftR : PMIOPort  Port=8  Side=Right
  CircleShiftCyl : PMIOPort  Port=9  Side=Right
  Out Bus Element : Outport  PortName=m  Element=LiftL
  Out Bus Element1 : Outport  PortName=m  Element=LiftR
  Out Bus Element2 : Outport  PortName=m  Element=CircleShift
  Out Bus Element3 : Outport  PortName=m  Element=LinkBar
  wires:
  Bus Element In/1 -> Saddle L/1(cmd)
  Bus Element In1/1 -> Circle Shift/1(cmd)
  Bus Element In2/1 -> Saddle R/1(cmd)
  Bus Element In3/1 -> LinkBar/1(cmd)
  Saddle L/1(m) -> Out Bus Element/1
  Saddle R/1(m) -> Out Bus Element1/1
  Circle Shift/1(m) -> Out Bus Element2/1
  LinkBar/1(m) -> Out Bus Element3/1
  connections:
  Saddle L/LConn2 -- LiftL/RConn1
  Saddle L/RConn1 -- FrameL/RConn1
  Saddle R/RConn2 -- LinkBar/LConn1
  LiftR/RConn1 -- Saddle R/LConn2
  FrameR/RConn1 -- Saddle R/RConn1
  Circle Shift/RConn1 -- Saddle L/RConn3
  CircleShiftCyl/RConn1 -- Circle Shift/LConn2
  LinkBar/RConn1 -- Saddle L/RConn2
  Pin/RConn1 -- LinkBar/LConn2
  Circle/RConn1 -- Circle Shift/LConn1
  LiftLR/RConn1 -- Saddle L/LConn1
  LiftRR/RConn1 -- Saddle R/LConn1

== system sm_motor_grader_lib/Position ==
  pCmd : Inport
  pMeas : Inport  Port=2
  Terminator : Terminator
  Terminator1 : Terminator
  R : PMIOPort  Side=Right
  wires:
  pMeas/1 -> Terminator1/1
  pCmd/1 -> Terminator/1

== system sm_motor_grader_lib/Powertrain ==
  Cmd : Inport
  m : Inport  Port=2
  CVT : Subsystem  VariantControl=CVT
      settings: PortSchema="{\"entries\":[{\"content\":{\"sides\":[{\"content\":{\"connectorIds\":[\"In1\",\"In2\"]},\"type\":\"ConnectorPlacement.EquallySpacedRectSide\",\"uuid\":\"b0ddd375-51b8-44b6-b073-16b56860cf73\"},{\"content\":{\"connectorIds\":[\"RConn1\",\"Out1\"],\"side\":\"RIGHT\"},\"type\":\"ConnectorPlacement.EquallySpacedRectSide\",\"uuid\":\"f6b94886-5d75-4a34-bd54-ed8eca8a2f91\"},{\"content\":{\"side\":\"TOP\"},\"type\":\"ConnectorPlacement.EquallySpacedRectSide\",\"uuid\":\"a9bdb5f3-5bc9-4293-95f7-be33271ad817\"}]},\"type\":\"ConnectorPlacement.EquallySpacedConnector\",\"uuid\":\"99647ee7-7b0f-4a9d-8234-cdeac05b9707\"}],\"packageUris\":[\"http://schema.mathworks.com/mf0/Connector/R2020b\"],\"version\":\"1.0\"}"
      mask Display: image('ssc_4whl_powertrain_cvt.png')
  Torque1 : Subsystem  VariantControl=Torque1
      settings: PortSchema="{\"entries\":[{\"content\":{\"sides\":[{\"content\":{\"connectorIds\":[\"In1\",\"In2\"]},\"type\":\"ConnectorPlacement.EquallySpacedRectSide\",\"uuid\":\"b0ddd375-51b8-44b6-b073-16b56860cf73\"},{\"content\":{\"connectorIds\":[\"RConn1\",\"Out1\"],\"side\":\"RIGHT\"},\"type\":\"ConnectorPlacement.EquallySpacedRectSide\",\"uuid\":\"f6b94886-5d75-4a34-bd54-ed8eca8a2f91\"},{\"content\":{\"side\":\"TOP\"},\"type\":\"ConnectorPlacement.EquallySpacedRectSide\",\"uuid\":\"a9bdb5f3-5bc9-4293-95f7-be33271ad817\"}]},\"type\":\"ConnectorPlacement.EquallySpacedConnector\",\"uuid\":\"99647ee7-7b0f-4a9d-8234-cdeac05b9707\"}],\"packageUris\":[\"http://schema.mathworks.com/mf0/Connector/R2020b\"],\"version\":\"1.0\"}"
      mask Display: image('ssc_4whl_powertrain_torque1.png')
  Torque4 : Subsystem  VariantControl=Torque4
      settings: PortSchema="{\"entries\":[{\"content\":{\"sides\":[{\"content\":{\"connectorIds\":[\"In1\",\"In2\"]},\"type\":\"ConnectorPlacement.EquallySpacedRectSide\",\"uuid\":\"b0ddd375-51b8-44b6-b073-16b56860cf73\"},{\"content\":{\"connectorIds\":[\"RConn1\",\"Out1\"],\"side\":\"RIGHT\"},\"type\":\"ConnectorPlacement.EquallySpacedRectSide\",\"uuid\":\"f6b94886-5d75-4a34-bd54-ed8eca8a2f91\"},{\"content\":{\"side\":\"TOP\"},\"type\":\"ConnectorPlacement.EquallySpacedRectSide\",\"uuid\":\"a9bdb5f3-5bc9-4293-95f7-be33271ad817\"}]},\"type\":\"ConnectorPlacement.EquallySpacedConnector\",\"uuid\":\"99647ee7-7b0f-4a9d-8234-cdeac05b9707\"}],\"packageUris\":[\"http://schema.mathworks.com/mf0/Connector/R2020b\"],\"version\":\"1.0\"}"
      mask Display: image('ssc_4whl_powertrain_torque4.png')
  Dtr : PMIOPort  Side=Right
  meas : Outport

== system sm_motor_grader_lib/Shaft ==
  pCmd : Inport
  pMeas : Inport  Port=2
  Force Source : fl_lib/Mechanical/Mechanical Sources/Ideal Force Source
  Gain : Gain  Gain=Kp
  Gain1 : Gain  Gain=Ki
  Gain2 : Gain  Gain=Kd
  Integrator : Integrator
  Mechanical Translational Reference2 : fl_lib/Mechanical/Translational Elements/Mechanical Translational Reference
  Simulink-PS Converter2 : nesl_utility/Simulink-PS Converter  PhysicalDomain=network_engine_domain  SubClassName=ps_input  LeftPortType=input  RightPortType=output  PseudoPeriodic=off  Frequencies=[]  NoiseDistribution=none  NoiseParameters=[]  Unit=1  AffineConversion=off  FilteringAndDerivatives=provide  SimscapeFilterOrder=1  InputFilterTimeConstant=0.001  UdotUserProvided=0
  Subtract : Sum  Inputs=+-
  Sum1 : Sum  Inputs=+++
  Transfer Fcn : TransferFcn  Numerator=[1 0]  Denominator=[0.01 1]
  Transfer Fcn (with initial outputs) : simulink_extras/Additional Linear/Transfer Fcn (with initial outputs)  N=[1]  D="[0.01  1]"  Y0=p_init  U0=p_init
  R : PMIOPort  Side=Right
  wires:
  Integrator/1 -> Sum1/2
  Gain/1 -> Sum1/1
  Transfer Fcn (with initial outputs)/1 -> Subtract/2
  Sum1/1 -> Simulink-PS Converter2/1  "Force Command"
  pMeas/1 -> Transfer Fcn (with initial outputs)/1
  pCmd/1 -> Subtract/1
  Gain1/1 -> Integrator/1
  Gain2/1 -> Transfer Fcn/1
  Subtract/1 -> Gain2/1, Gain1/1, Gain/1
  Transfer Fcn/1 -> Sum1/3
  connections:
  Force Source/RConn2 -- Mechanical Translational Reference2/LConn1
  Simulink-PS Converter2/RConn1 -- Force Source/RConn1
  R/RConn1 -- Force Source/LConn1
